simulink model "base_1fm"  (R2016b)
settings: Solver=FixedStepDiscrete  StartTime=0.0  StopTime=inf  FixedStep=sampleTime  RelTol=1e-3
InitFcn:
  | base_1fm_parameters;
StartFcn:
  | base_1fm_parameters;
values from neighbouring files (symbols this model uses):
  Lb = 0.07    [base_1fm_parameters.m]    (also in parameters_base_model_bros.m)
  Lf = 0.238    [base_1fm_parameters.m]    (also in parameters_base_model_bros.m)
  Lu = 0.153    [base_1fm_parameters.m]    (also in parameters_base_model_bros.m)
  sampleTime = 0.001    [base_1fm_parameters.m]    (also in parameters_base_model_bros.m)
undefined symbols (not defined in the file or in its folder): FM1
libraries: simulink x5, LibraryFM x1, FMLibrary_v2 x1
settings Model: SimulationMode=external  Creator=niekbeckers  LastModifiedBy=Labuser
settings DataIOCC: LimitDataPoints=on  SaveFormat=Array
settings OptimizationCC: BlockReduction=off  BooleanDataType=off  LocalBlockOutputs=off  LifeSpan=inf
settings DebuggingCC: SaveWithParameterizedLinksMsg=none  UnderspecifiedInitializationDetection=Classic  MergeDetectMultiDrivingBlocksExec=none  SignalResolutionControl=TryResolveAllWithWarning  SFUnexpectedBacktrackingDiag=warning  SFNoUnconditionalDefaultTransitionDiag=warning  SFExecutionAtInitializationDiag=none
settings HardwareCC: ProdBitPerPointer=32  ProdBitPerSizeT=32  ProdBitPerPtrDiffT=32  ProdLargestAtomicFloat=None  ProdIntDivRoundTo=Undefined  ProdEndianess=Unspecified  ProdWordSize=32  ProdHWDeviceType=32-bit Generic  TargetBitPerPointer=64  TargetBitPerSizeT=64  TargetBitPerPtrDiffT=64  TargetLongLongMode=on  TargetIntDivRoundTo=Zero  TargetEndianess=LittleEndian  TargetWordSize=64  TargetHWDeviceType=MATLAB Host  ProdEqTarget=off
settings ModelReferenceCC: PropagateSignalLabelsOutOfModel=off
settings RTWCC: SystemTargetFile=TwinCAT.tlc  GenCodeOnly=on  MakeCommand=make_tct  TemplateMakefile=tct_msbuild.tmf  Description=TwinCAT Target  GenerateReport=on  TargetLang=C++
settings STFCustomTargetCC: CompOptLevelCompliant=on  GeneratePreprocessorConditionals=Disable all  MATLABClassNameForMDSCustomization=Simulink.SoftwareTarget.TargetSpecificTriggerConfigurationBase  SystemTargetFile=TwinCAT.tlc
settings ConfigComp: CovMetricSettings=dw  CovHtmlReporting=on  CovSaveCumulativeToWorkspaceVar=on  CovSaveSingleToWorkspaceVar=on  CovExternalEMLEnable=off  CovSFcnEnable=off

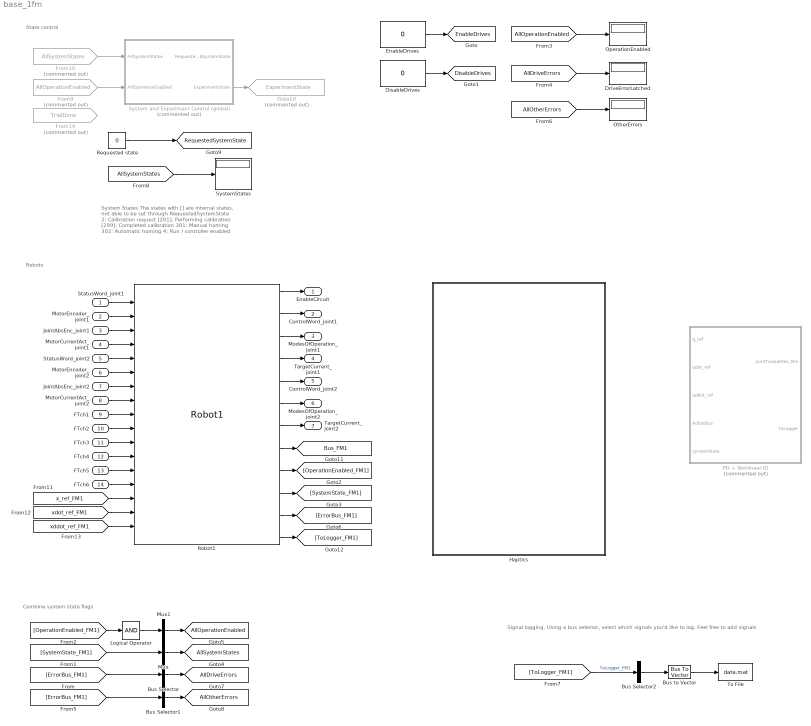
== system base_1fm ==
  note: Signal logging.
      | Using a bus selector, select which signals you'd like to log. Feel free to add signals
  note: System States
      | The states with [] are internal states, not able to be set through RequestedSystemState
      | 2: Calibration request
      | [201]: Performing calibration
      | [299]: Completed calibration
      | 301: Manual homing
      | 302: Automatic homing
      | 4: Run / controller enabled
  note: State control
  note: Combine system state flags
  note: Robots
  StatusWord_joint1 : Inport  OutDataTypeStr=uint16  PortDimensions=1
  MotorEncoder_joint1 : Inport  Port=2  OutDataTypeStr=int32  PortDimensions=1
  JointAbsEnc_joint1 : Inport  Port=3  OutDataTypeStr=int32  PortDimensions=1
  MotorCurrentAct_joint1 : Inport  Port=4  OutDataTypeStr=int16  PortDimensions=1
  StatusWord_joint2 : Inport  Port=5  OutDataTypeStr=uint16  PortDimensions=1
  MotorEncoder_joint2 : Inport  Port=6  OutDataTypeStr=int32  PortDimensions=1
  JointAbsEnc_joint2 : Inport  Port=7  OutDataTypeStr=int32  PortDimensions=1
  MotorCurrentAct_joint2 : Inport  Port=8  OutDataTypeStr=int16  PortDimensions=1
  FTch1 : Inport  Port=9  OutDataTypeStr=single  PortDimensions=1
  FTch2 : Inport  Port=10  OutDataTypeStr=single  PortDimensions=1
  FTch3 : Inport  Port=11  OutDataTypeStr=single  PortDimensions=1
  FTch4 : Inport  Port=12  OutDataTypeStr=single  PortDimensions=1
  FTch5 : Inport  Port=13  OutDataTypeStr=single  PortDimensions=1
  FTch6 : Inport  Port=14  OutDataTypeStr=single  PortDimensions=1
  Bus Selector : BusSelector  OutputSignals=DriveErrorLatched  OutputAsBus=on
  Bus Selector1 : BusSelector  OutputSignals=WorkspaceErrorLatched,ForceSensorLatched  OutputAsBus=on
  Bus Selector2 : BusSelector  OutputSignals=SystemState,ToLogger_ToEtherCAT.ToLogger_Actuator1.JointPosition_rad,ToLogger_ToEtherCAT.ToLogger_Actuator1.JointVelocity_rads,ToLogger_ToEtherCAT.ToLogger_Actuator1.JointTorque_Act_Nm,ToLogger_ToEtherCAT.ToLogger_Actuator1.DesiredTorqueLimited_Nm,ToLogger_ToEtherCAT.ToLogger_Actuator1.DriveError,ToLogger_ToEtherCAT.ToLogger_Actuator2.JointPosition_rad,ToLogger_ToEtherCAT.ToLogger_Actuator2.JointVelocity_rads,ToLogger_ToEtherCAT.ToLogger_Actuator2.JointTorque_Act_Nm,ToLogger_ToEtherCAT.ToLogger_Actuator2.DesiredTorqueLimited_Nm,ToLogger_ToEtherCAT.ToLogger_Actuator2.DriveError,ToLogger_Controller.q_ref,ToLogger_Controller.qdot_ref,ToLogger_Controller.qddot_ref  OutputAsBus=on
  Bus to Vector : BusToVector
  DisableDrives : Constant  Value=0
      settings: OpenFcn=set_param(gcb,'Value','1');tname = ['toggletimer_' gcb];delete(timerfind('name',tname));t = timer('timerfcn', ['set_param(''',gcb,''',''Value'',''0'')'],'executionmode','singleshot','startdelay',1,'name',tname);start(t);
      mask Display: fprintf('PushToTrigger\n%s',get_param(gcb,'value'))
  DriveErrorLatched : Display
  EnableDrives : Constant  Value=0
      settings: OpenFcn=set_param(gcb,'Value','1');tname = ['toggletimer_' gcb];delete(timerfind('name',tname));t = timer('timerfcn', ['set_param(''',gcb,''',''Value'',''0'')'],'executionmode','singleshot','startdelay',1,'name',tname);start(t);
      mask Display: fprintf('PushToTrigger\n%s',get_param(gcb,'value'))
  From10 : From  Commented=on  GotoTag=AllSystemStates
  From14 : From  Commented=on  GotoTag=TrialDone
  From9 : From  Commented=on  GotoTag=AllOperationEnabled
  Goto10 : Goto  Commented=on  GotoTag=ExperimentState  TagVisibility=global
  Haptics : Subsystem
  Logical Operator : Logic  Inputs=1  AllPortsSameDT=off  OutDataTypeStr=boolean
  Mux : Mux  Inputs=1
  Mux1 : Mux  Inputs=1
  OperationEnabled : Display
  OtherErrors : Display
  PD + Nonlinear ID : Subsystem  Commented=on  AncestorBlock=LibraryFM/Robot1/Controller/PD + Nonlinear ID
  Requested state : Constant  Value=0
  Robot1 : LibraryFM/Robot1  RobotStruct=FM1
  System and Experiment Control (global) : Subsystem  Commented=on
  SystemStates : Display
  To File : ToFile  Filename=data.mat
  EnableCircuit : Outport  OutDataTypeStr=boolean  PortDimensions=1
  ControlWord_joint1 : Outport  Port=2  OutDataTypeStr=uint16  PortDimensions=1
  ModesOfOperation_joint1 : Outport  Port=3  OutDataTypeStr=int8  PortDimensions=1
  TargetCurrent_joint1 : Outport  Port=4  OutDataTypeStr=int16  PortDimensions=1
  ControlWord_joint2 : Outport  Port=5  OutDataTypeStr=uint16  PortDimensions=1
  ModesOfOperation_joint2 : Outport  Port=6  OutDataTypeStr=int8  PortDimensions=1
  TargetCurrent_joint2 : Outport  Port=7  OutDataTypeStr=int16  PortDimensions=1
  tag scope: AllDriveErrors=global, AllOperationEnabled=global, AllOtherErrors=global, AllSystemStates=global, Bus_FM1=global, DisableDrives=global, EnableDrives=global, RequestedSystemState=global
  wires:
  DisableDrives/1 -> [DisableDrives]
  EnableDrives/1 -> [EnableDrives]
  Robot1/9 -> [OperationEnabled_FM1]
  [AllOperationEnabled] -> OperationEnabled/1
  Robot1/10 -> [SystemState_FM1]
  [SystemState_FM1] -> Mux/1
  Mux/1 -> [AllSystemStates]
  Mux1/1 -> [AllOperationEnabled]
  [OperationEnabled_FM1] -> Logical Operator/1
  Robot1/11 -> [ErrorBus_FM1]
  [ErrorBus_FM1] -> Bus Selector/1
  Bus Selector/1 -> [AllDriveErrors]
  [AllDriveErrors] -> DriveErrorLatched/1
  [ErrorBus_FM1] -> Bus Selector1/1
  Bus Selector1/1 -> [AllOtherErrors]
  [AllOtherErrors] -> OtherErrors/1
  [AllSystemStates] -> SystemStates/1
  System and Experiment Control (global)/2(ExperimentState) -> Goto10/1
  From10/1 -> System and Experiment Control (global)/1(AllSystemStates)
  From9/1 -> System and Experiment Control (global)/2(AllOperationEnabled)
  [x_ref_FM1] -> Robot1/15
  [xdot_ref_FM1] -> Robot1/16
  [xddot_ref_FM1] -> Robot1/17
  Requested state/1 -> [RequestedSystemState]
  Robot1/8 -> [Bus_FM1]
  StatusWord_joint1/1 -> Robot1/1
  MotorEncoder_joint1/1 -> Robot1/2
  JointAbsEnc_joint1/1 -> Robot1/3
  MotorCurrentAct_joint1/1 -> Robot1/4
  StatusWord_joint2/1 -> Robot1/5
  MotorEncoder_joint2/1 -> Robot1/6
  JointAbsEnc_joint2/1 -> Robot1/7
  MotorCurrentAct_joint2/1 -> Robot1/8
  FTch1/1 -> Robot1/9
  FTch2/1 -> Robot1/10
  FTch3/1 -> Robot1/11
  FTch4/1 -> Robot1/12
  FTch5/1 -> Robot1/13
  FTch6/1 -> Robot1/14
  Robot1/1 -> EnableCircuit/1
  Robot1/2 -> ControlWord_joint1/1
  Robot1/3 -> ModesOfOperation_joint1/1
  Robot1/4 -> TargetCurrent_joint1/1
  Robot1/7 -> TargetCurrent_joint2/1
  Robot1/6 -> ModesOfOperation_joint2/1
  Robot1/5 -> ControlWord_joint2/1
  Robot1/12 -> [ToLogger_FM1]
  [ToLogger_FM1] -> Bus Selector2/1  "ToLogger_FM1"
  Bus Selector2/1 -> Bus to Vector/1
  Bus to Vector/1 -> To File/1
  Logical Operator/1 -> Mux1/1

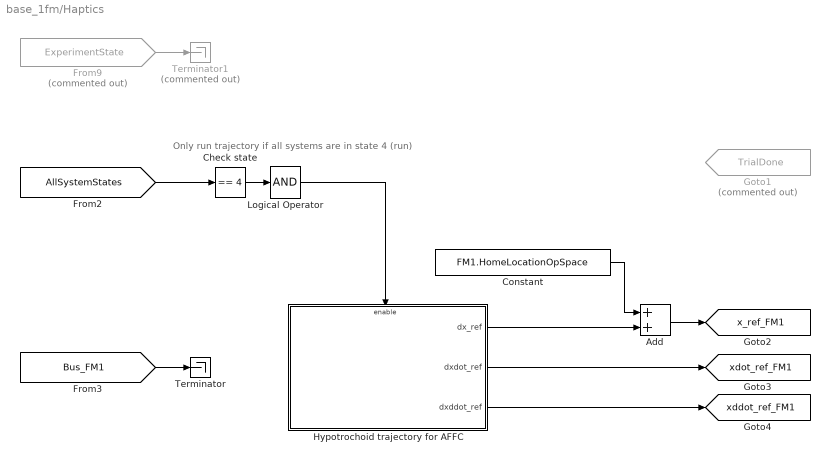
== system base_1fm/Haptics ==
  note: Only run trajectory if all systems are in state 4 (run)
  Add : Sum
  "Check state " : simulink/Logic and Bit Operations/Compare To Constant  relop===  const=4  OutDataTypeStr=boolean
  Constant : Constant  Value=FM1.HomeLocationOpSpace
  From9 : From  Commented=on  GotoTag=ExperimentState
  Goto1 : Goto  Commented=on  GotoTag=TrialDone  TagVisibility=global
  Hypotrochoid trajectory for AFFC : Subsystem
  Logical Operator : Logic  Inputs=1  AllPortsSameDT=off  OutDataTypeStr=boolean
  Terminator : Terminator
  Terminator1 : Terminator  Commented=on
  tag scope: x_ref_FM1=global, xddot_ref_FM1=global, xdot_ref_FM1=global
  wires:
  [Bus_FM1] -> Terminator/1
  Constant/1 -> Add/1
  Hypotrochoid trajectory for AFFC/1(dx_ref) -> Add/2
  Add/1 -> [x_ref_FM1]
  Hypotrochoid trajectory for AFFC/2(dxdot_ref) -> [xdot_ref_FM1]
  Hypotrochoid trajectory for AFFC/3(dxddot_ref) -> [xddot_ref_FM1]
  [AllSystemStates] -> "Check state "/1
  "Check state "/1 -> Logical Operator/1
  Logical Operator/1 -> Hypotrochoid trajectory for AFFC/Enable
  From9/1 -> Terminator1/1

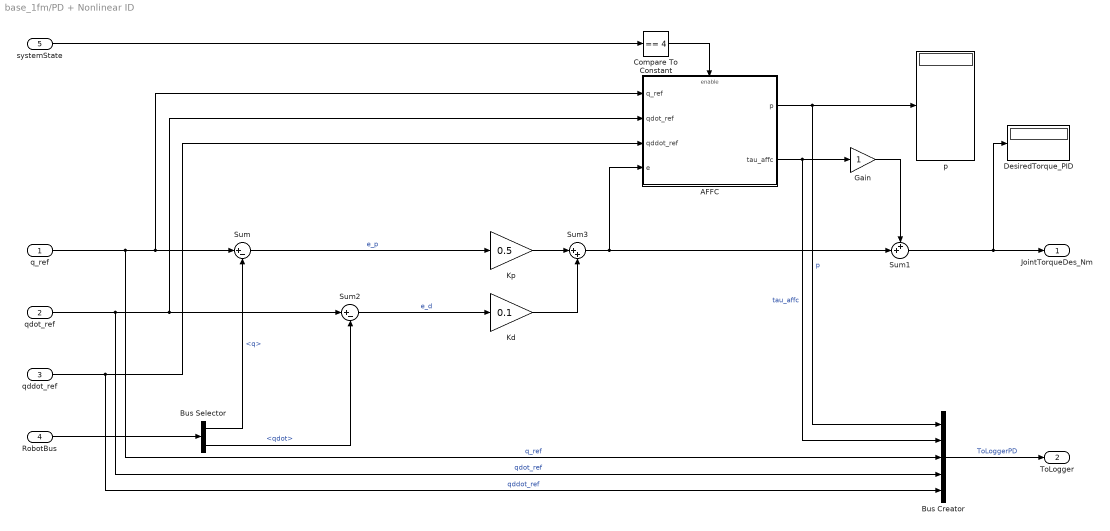
== system base_1fm/PD + Nonlinear ID ==
  q_ref : Inport
  qdot_ref : Inport  Port=2
  qddot_ref : Inport  Port=3
  RobotBus : Inport  Port=4
  systemState : Inport  Port=5
  AFFC : Subsystem
  Bus Creator : BusCreator  Inputs=5
  Bus Selector : BusSelector  OutputSignals=qJointSpace.q,qJointSpace.qdot
  Compare To Constant : simulink/Logic and Bit Operations/Compare To Constant  relop===  const=4  OutDataTypeStr=boolean
  DesiredTorque_PID : Display
  Gain : Gain
  Kd : Gain  Gain=0.1
  Kp : Gain  Gain=0.5
  Sum : Sum  Inputs=|+-
  Sum1 : Sum  Inputs=++|
  Sum2 : Sum  Inputs=|+-
  Sum3 : Sum  Inputs=|++
  p : Display
  JointTorqueDes_Nm : Outport
  ToLogger : Outport  Port=2
  wires:
  Bus Selector/2 -> Sum2/2  "<qdot>"
  Bus Selector/1 -> Sum/2  "<q>"
  q_ref/1 -> Bus Creator/3, AFFC/1(q_ref), Sum/1  "q_ref"
  Sum/1 -> Kp/1  "e_p"
  Sum3/1 -> AFFC/4(e), Sum1/2
  Kd/1 -> Sum3/2
  Kp/1 -> Sum3/1
  qdot_ref/1 -> Bus Creator/4, AFFC/2(qdot_ref), Sum2/1  "qdot_ref"
  Sum2/1 -> Kd/1  "e_d"
  Gain/1 -> Sum1/1
  Sum1/1 -> JointTorqueDes_Nm/1, DesiredTorque_PID/1
  RobotBus/1 -> Bus Selector/1
  qddot_ref/1 -> Bus Creator/5, AFFC/3(qddot_ref)  "qddot_ref"
  AFFC/1(p) -> Bus Creator/1, p/1  "p"
  AFFC/2(tau_affc) -> Bus Creator/2, Gain/1  "tau_affc"
  systemState/1 -> Compare To Constant/1
  Compare To Constant/1 -> AFFC/Enable
  Bus Creator/1 -> ToLogger/1  "ToLoggerPD"

== system base_1fm/System and Experiment Control (global) ==
  note: Hier ergens experiment protocol inlezen
  AllSystemStates : Inport
  AllOperationEnabled : Inport  Port=2
  GlobalStateMachine : FMLibrary_v2/StateMachineLocal/SystemLocalStateMachine
  RequestedSystemState : Outport
  ExperimentState : Outport  Port=2
  wires:
  GlobalStateMachine/1 -> RequestedSystemState/1

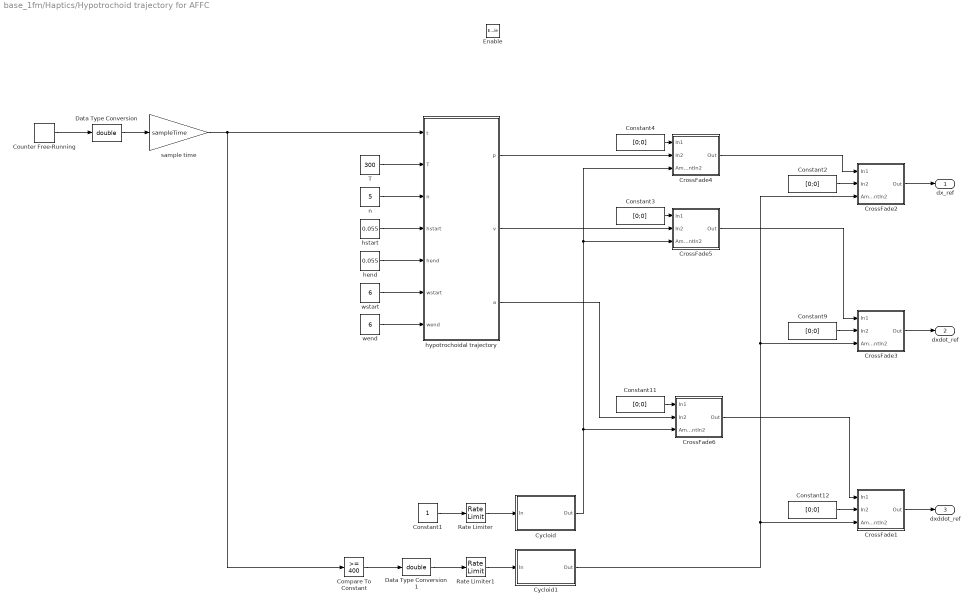
== system base_1fm/Haptics/Hypotrochoid trajectory for AFFC ==
  Enable : EnablePort  StatesWhenEnabling=reset
  Compare To Constant : simulink/Logic and Bit Operations/Compare To Constant  relop=>=  const=400  OutDataTypeStr=boolean
  Constant1 : Constant
  Constant{2..4,9,11..12} (6 alike) : Constant  Value=[0;0]
  Counter Free-Running : simulink/Sources/Counter Free-Running  NumBits=32  tsamp=-1
  CrossFade1 : Subsystem  AncestorBlock=VariousBlocksLibrary/Various/CrossFade
  CrossFade2 : Subsystem  AncestorBlock=VariousBlocksLibrary/Various/CrossFade
  CrossFade3 : Subsystem  AncestorBlock=VariousBlocksLibrary/Various/CrossFade
  CrossFade4 : Subsystem
  CrossFade5 : Subsystem  AncestorBlock=VariousBlocksLibrary/Various/CrossFade
  CrossFade6 : Subsystem  AncestorBlock=VariousBlocksLibrary/Various/CrossFade
  Cycloid : Subsystem  AncestorBlock=VariousBlocksLibrary/Various/Cycloid
  Cycloid1 : Subsystem  AncestorBlock=VariousBlocksLibrary/Various/Cycloid
  Data Type Conversion : DataTypeConversion  OutDataTypeStr=double
  Data Type Conversion1 : DataTypeConversion  OutDataTypeStr=double
  Rate Limiter : RateLimiter  RisingSlewLimit=0.25  FallingSlewLimit=-0.15  SampleTimeMode=inherited
  Rate Limiter1 : RateLimiter  RisingSlewLimit=0.2  FallingSlewLimit=-0.2  SampleTimeMode=inherited
  T : Constant  Value=300
  hend : Constant  Value=0.055
  hstart : Constant  Value=0.055
  hypotrochoidal trajectory : MATLAB Function  TreatAsAtomicUnit=on
  n : Constant  Value=5
  sample time : Gain  Gain=sampleTime
  wend : Constant  Value=6
  wstart : Constant  Value=6
  dx_ref : Outport
  dxdot_ref : Outport  Port=2
  dxddot_ref : Outport  Port=3
  wires:
  Data Type Conversion1/1 -> Rate Limiter1/1
  hypotrochoidal trajectory/1(p) -> CrossFade4/2(In2)
  CrossFade1/1(Out) -> dxddot_ref/1
  Constant11/1 -> CrossFade6/1(In1)
  Constant12/1 -> CrossFade1/2(In2)
  CrossFade6/1(Out) -> CrossFade1/1(In1)
  Constant9/1 -> CrossFade3/2(In2)
  CrossFade5/1(Out) -> CrossFade3/1(In1)
  CrossFade3/1(Out) -> dxdot_ref/1
  Cycloid1/1(Out) -> CrossFade1/3(AmountIn2), CrossFade2/3(AmountIn2), CrossFade3/3(AmountIn2)
  Rate Limiter1/1 -> Cycloid1/1(In)
  Compare To Constant/1 -> Data Type Conversion1/1
  CrossFade4/1(Out) -> CrossFade2/1(In1)
  CrossFade2/1(Out) -> dx_ref/1
  Rate Limiter/1 -> Cycloid/1(In)
  Constant1/1 -> Rate Limiter/1
  Cycloid/1(Out) -> CrossFade6/3(AmountIn2), CrossFade5/3(AmountIn2), CrossFade4/3(AmountIn2)
  hypotrochoidal trajectory/2(v) -> CrossFade5/2(In2)
  hypotrochoidal trajectory/3(a) -> CrossFade6/2(In2)
  sample time/1 -> Compare To Constant/1, hypotrochoidal trajectory/1(t)
  Constant2/1 -> CrossFade2/2(In2)
  Data Type Conversion/1 -> sample time/1
  wstart/1 -> hypotrochoidal trajectory/6(wstart)
  wend/1 -> hypotrochoidal trajectory/7(wend)
  hstart/1 -> hypotrochoidal trajectory/4(hstart)
  hend/1 -> hypotrochoidal trajectory/5(hend)
  n/1 -> hypotrochoidal trajectory/3(n)
  T/1 -> hypotrochoidal trajectory/2(T)
  Counter Free-Running/1 -> Data Type Conversion/1
  Constant3/1 -> CrossFade5/1(In1)
  Constant4/1 -> CrossFade4/1(In1)

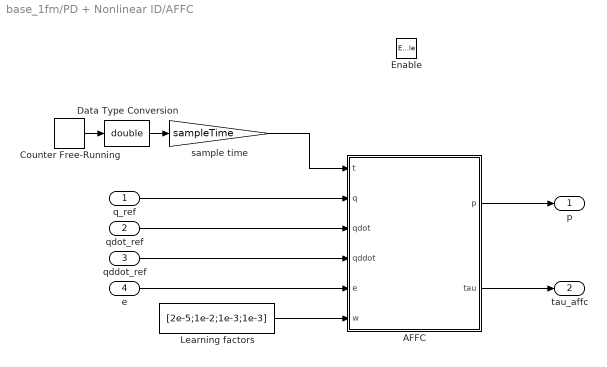
== system base_1fm/PD + Nonlinear ID/AFFC ==
  q_ref : Inport
  qdot_ref : Inport  Port=2
  qddot_ref : Inport  Port=3
  e : Inport  Port=4
  Enable : EnablePort  StatesWhenEnabling=reset
  AFFC : MATLAB Function  TreatAsAtomicUnit=on
  Counter Free-Running : simulink/Sources/Counter Free-Running  NumBits=32  tsamp=-1
  Data Type Conversion : DataTypeConversion  OutDataTypeStr=double
  Learning factors : Constant  Value=[2e-5;1e-2;1e-3;1e-3]
  sample time : Gain  Gain=sampleTime
  p : Outport  OutputWhenDisabled=reset
  tau_affc : Outport  Port=2  OutputWhenDisabled=reset  InitialOutput=[0;0]
  wires:
  Learning factors/1 -> AFFC/6(w)
  Data Type Conversion/1 -> sample time/1
  sample time/1 -> AFFC/1(t)
  Counter Free-Running/1 -> Data Type Conversion/1
  AFFC/1(p) -> p/1
  AFFC/2(tau) -> tau_affc/1
  q_ref/1 -> AFFC/2(q)
  qdot_ref/1 -> AFFC/3(qdot)
  qddot_ref/1 -> AFFC/4(qddot)
  e/1 -> AFFC/5(e)

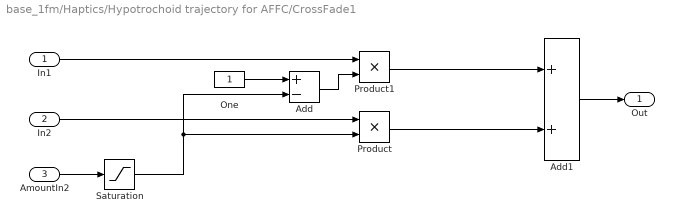
== system base_1fm/Haptics/Hypotrochoid trajectory for AFFC/CrossFade1 ==
  In1 : Inport
  In2 : Inport  Port=2
  AmountIn2 : Inport  Port=3
  Add : Sum  Inputs=+-
  Add1 : Sum
  One : Constant
  Product : Product  RndMeth=Zero
  Product1 : Product  RndMeth=Zero
  Saturation : Saturate  UpperLimit=1  LowerLimit=0
  Out : Outport
  wires:
  In1/1 -> Product1/1
  AmountIn2/1 -> Saturation/1
  One/1 -> Add/1
  Saturation/1 -> Product/2, Add/2
  Add/1 -> Product1/2
  Product/1 -> Add1/2
  Product1/1 -> Add1/1
  In2/1 -> Product/1
  Add1/1 -> Out/1

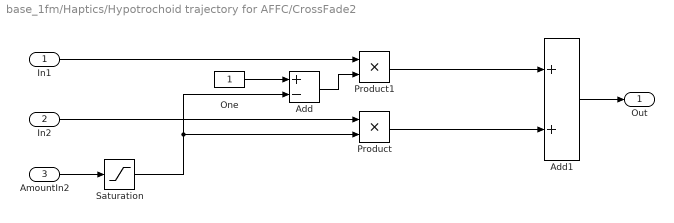
== system base_1fm/Haptics/Hypotrochoid trajectory for AFFC/CrossFade2 ==
  In1 : Inport
  In2 : Inport  Port=2
  AmountIn2 : Inport  Port=3
  Add : Sum  Inputs=+-
  Add1 : Sum
  One : Constant
  Product : Product  RndMeth=Zero
  Product1 : Product  RndMeth=Zero
  Saturation : Saturate  UpperLimit=1  LowerLimit=0
  Out : Outport
  wires:
  In1/1 -> Product1/1
  AmountIn2/1 -> Saturation/1
  One/1 -> Add/1
  Saturation/1 -> Product/2, Add/2
  Add/1 -> Product1/2
  Product/1 -> Add1/2
  Product1/1 -> Add1/1
  In2/1 -> Product/1
  Add1/1 -> Out/1

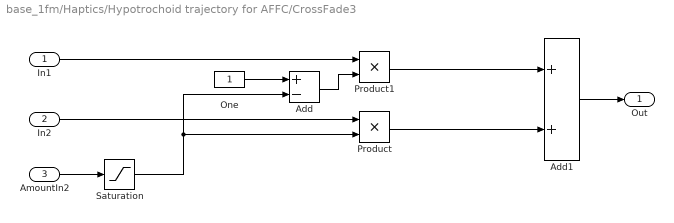
== system base_1fm/Haptics/Hypotrochoid trajectory for AFFC/CrossFade3 ==
  In1 : Inport
  In2 : Inport  Port=2
  AmountIn2 : Inport  Port=3
  Add : Sum  Inputs=+-
  Add1 : Sum
  One : Constant
  Product : Product  RndMeth=Zero
  Product1 : Product  RndMeth=Zero
  Saturation : Saturate  UpperLimit=1  LowerLimit=0
  Out : Outport
  wires:
  In1/1 -> Product1/1
  AmountIn2/1 -> Saturation/1
  One/1 -> Add/1
  Saturation/1 -> Product/2, Add/2
  Add/1 -> Product1/2
  Product/1 -> Add1/2
  Product1/1 -> Add1/1
  In2/1 -> Product/1
  Add1/1 -> Out/1

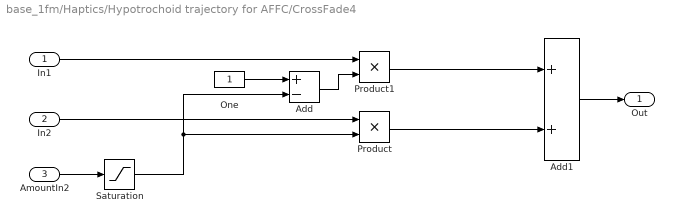
== system base_1fm/Haptics/Hypotrochoid trajectory for AFFC/CrossFade4 ==
  In1 : Inport
  In2 : Inport  Port=2
  AmountIn2 : Inport  Port=3
  Add : Sum  Inputs=+-
  Add1 : Sum
  One : Constant
  Product : Product  RndMeth=Zero
  Product1 : Product  RndMeth=Zero
  Saturation : Saturate  UpperLimit=1  LowerLimit=0
  Out : Outport
  wires:
  In1/1 -> Product1/1
  AmountIn2/1 -> Saturation/1
  One/1 -> Add/1
  Saturation/1 -> Product/2, Add/2
  Add/1 -> Product1/2
  Product/1 -> Add1/2
  Product1/1 -> Add1/1
  In2/1 -> Product/1
  Add1/1 -> Out/1

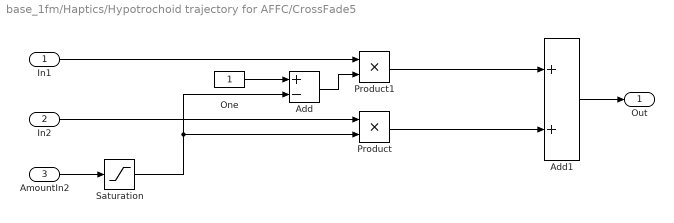
== system base_1fm/Haptics/Hypotrochoid trajectory for AFFC/CrossFade5 ==
  In1 : Inport
  In2 : Inport  Port=2
  AmountIn2 : Inport  Port=3
  Add : Sum  Inputs=+-
  Add1 : Sum
  One : Constant
  Product : Product  RndMeth=Zero
  Product1 : Product  RndMeth=Zero
  Saturation : Saturate  UpperLimit=1  LowerLimit=0
  Out : Outport
  wires:
  In1/1 -> Product1/1
  AmountIn2/1 -> Saturation/1
  One/1 -> Add/1
  Saturation/1 -> Product/2, Add/2
  Add/1 -> Product1/2
  Product/1 -> Add1/2
  Product1/1 -> Add1/1
  In2/1 -> Product/1
  Add1/1 -> Out/1

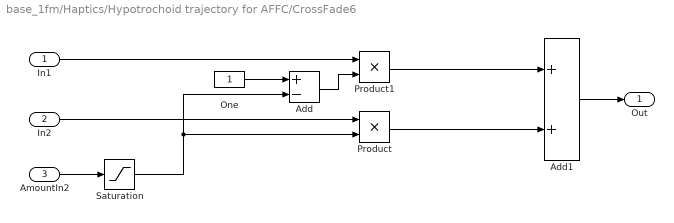
== system base_1fm/Haptics/Hypotrochoid trajectory for AFFC/CrossFade6 ==
  In1 : Inport
  In2 : Inport  Port=2
  AmountIn2 : Inport  Port=3
  Add : Sum  Inputs=+-
  Add1 : Sum
  One : Constant
  Product : Product  RndMeth=Zero
  Product1 : Product  RndMeth=Zero
  Saturation : Saturate  UpperLimit=1  LowerLimit=0
  Out : Outport
  wires:
  In1/1 -> Product1/1
  AmountIn2/1 -> Saturation/1
  One/1 -> Add/1
  Saturation/1 -> Product/2, Add/2
  Add/1 -> Product1/2
  Product/1 -> Add1/2
  Product1/1 -> Add1/1
  In2/1 -> Product/1
  Add1/1 -> Out/1

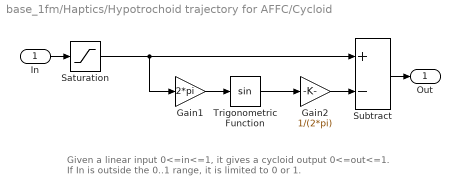
== system base_1fm/Haptics/Hypotrochoid trajectory for AFFC/Cycloid ==
  note: Given a linear input 0<=in<=1, it gives a cycloid output 0<=out<=1.
      | If In is outside the 0..1 range, it is limited to 0 or 1.
  In : Inport
  Gain1 : Gain  Gain=2*pi
  Gain2 : Gain  Gain=1/(2*pi)
  Saturation : Saturate  UpperLimit=1  LowerLimit=0
  Subtract : Sum  Inputs=+-
  Trigonometric Function : Trigonometry
  Out : Outport
  wires:
  Gain1/1 -> Trigonometric Function/1
  Subtract/1 -> Out/1
  In/1 -> Saturation/1
  Saturation/1 -> Gain1/1, Subtract/1
  Trigonometric Function/1 -> Gain2/1
  Gain2/1 -> Subtract/2

== system base_1fm/Haptics/Hypotrochoid trajectory for AFFC/Cycloid1 ==
  note: Given a linear input 0<=in<=1, it gives a cycloid output 0<=out<=1.
      | If In is outside the 0..1 range, it is limited to 0 or 1.
  In : Inport
  Gain1 : Gain  Gain=2*pi
  Gain2 : Gain  Gain=1/(2*pi)
  Saturation : Saturate  UpperLimit=1  LowerLimit=0
  Subtract : Sum  Inputs=+-
  Trigonometric Function : Trigonometry
  Out : Outport
  wires:
  Gain1/1 -> Trigonometric Function/1
  Subtract/1 -> Out/1
  In/1 -> Saturation/1
  Saturation/1 -> Gain1/1, Subtract/1
  Trigonometric Function/1 -> Gain2/1
  Gain2/1 -> Subtract/2

== matlab function base_1fm/PD + Nonlinear ID/AFFC/AFFC ==
  data: p output; t input; q input; qdot input; qddot input; e input; tau output; Lf parameter; Lu parameter; Lb parameter; w input
function [p,tau] = fcn(t, q, qdot, qddot, e, Lf, Lu, Lb,w)

persistent p_;

if isempty(p_)
%     p_ = [0.00173;0.00159;0.048;0.07889;-0.00389;0.08784;-0.00474];
    p_ = zeros(7,1);
end


% jacobians
J = func_eq_Je(q(1),q(2),Lf,Lu,Lb);
Jdot = func_eq_Jedot(q(1),q(2),qdot(1),qdot(2),Lf,Lu,Lb);

% create Psi
Psi = [diag([qddot(1) qddot(2)]) J'*J*qddot+J'*Jdot*qdot [sign(qdot(1)) qdot(1); 0 0] [0 0;sign(qdot(2)) qdot(2)] ];

% learning matrix Gamma
eta = 0.95*exp(-t/150) + 0.05;
% eta = 1;
% wI = 1e-3;
% wme = 5e-2;
% wfd = 1e-3;
% wfs = 1e-3;

wI = w(1);
wme = w(2);
wfd = w(3);
wfs = w(4);

Gamma = eta*diag([wI wI wme wfs wfd wfs wfd]);

% update p (parameter vector)
% learning rule
dp = Gamma*Psi'*e;
p_ = p_ + dp;

% Psi = [diag([qddot(1) qddot(2)]) J'*J*qddot+J'*Jdot*qdot [ssign(qdot(1)) qdot(1); 0 0] [0 0;ssign(qdot(2)) qdot(2)] ];

% feedforward torque
tau = Psi*p_;

p = p_;

function y = ssign(u,beta)
% soft sign
if nargin == 1
    beta = 150;
end

y = 2./(1+exp(-beta*u))-1;

== matlab function base_1fm/Haptics/Hypotrochoid trajectory for AFFC/hypotrochoidal trajectory ==
  data: t input; p output; v output; a output; T input; n input; hstart input; hend input; wstart input; wend input
function [p,v,a] = fcn(t,T,n,hstart,hend,wstart,wend)
%#codegen

p = func_p_hypothrochoid(t,T,n,hstart,hend,wstart,wend);
v = func_v_hypothrochoid(t,T,n,hstart,hend,wstart,wend);
a = func_a_hypothrochoid(t,T,n,hstart,hend,wstart,wend);
